simulink subsystem "No_Steering"  (R2025b)
settings: Solver=VariableStepAuto  StartTime=0.0  StopTime=10.0  RelTol=1e-3
undefined symbols (not defined in the file): InitStrAng
settings Model: Creator=The MathWorks, Inc.  LastModifiedBy=The MathWorks, Inc.
settings RTWCC: GPUComputeCapability=3.5

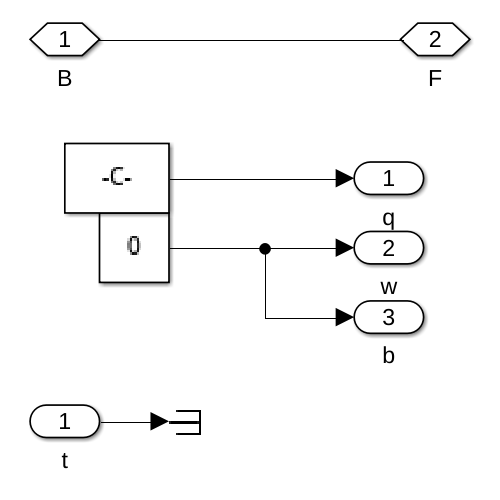
[thumbnail: Simulink's stored preview of the top-level diagram]
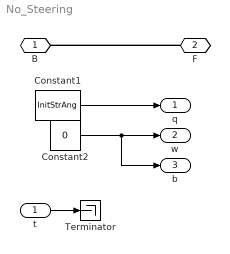
== system No_Steering ==
  t : Inport
  Constant1 : Constant  Value=InitStrAng
  Constant2 : Constant  Value=0
  Terminator : Terminator
  B : PMIOPort  Side=Left
  F : PMIOPort  Port=2  Side=Right
  q : Outport
  w : Outport  Port=2
  b : Outport  Port=3
  wires:
  Constant1/1 -> q/1
  Constant2/1 -> w/1, b/1
  t/1 -> Terminator/1
  connections:
  F/RConn1 -- B/RConn1
